simulink model "BPSK_Modulation"  (R2013a)
settings: Solver=ode3  StartTime=0.0  StopTime=0.06  FixedStep=1/(19200*2048)  RelTol=1e-3
libraries: simulink_extras x5, dsparch4 x2, simulink x1, commrandsrc2 x1
settings Model: Creator=Cedric  LastModifiedBy=Cedric
settings OptimizationCC: BooleanDataType=off

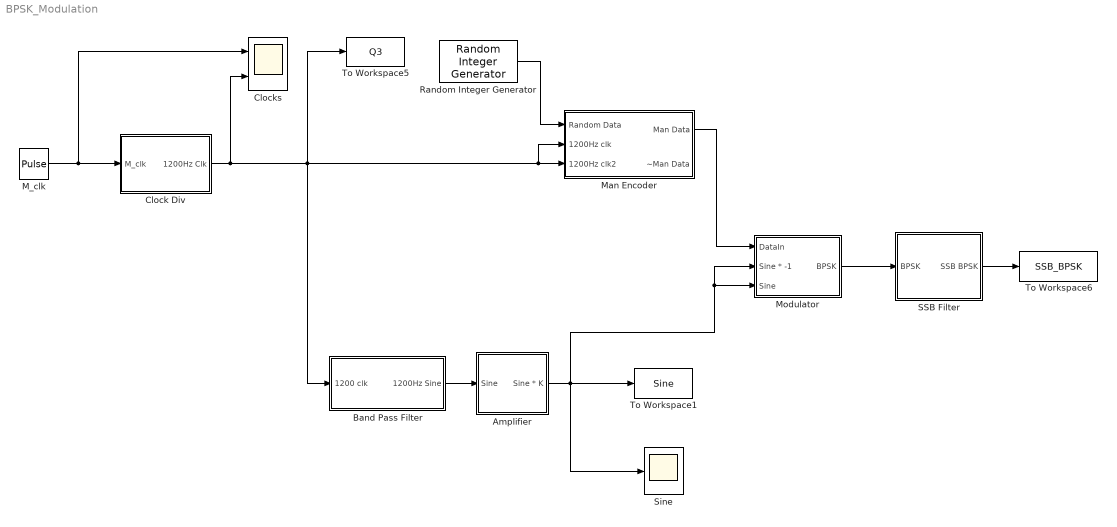
== system BPSK_Modulation ==
  Amplifier : Subsystem
  Band Pass Filter : Subsystem
  Clock Div : Subsystem
  Clocks : Scope  NumInputPorts=2
      settings: TimeRange=0.0003500000000000031  YMin=0~0  YMax=1~2
  M_clk : DiscretePulseGenerator  Period=4  PulseWidth=2  SampleTime=1/76800
  Man Encoder : Subsystem
  Modulator : Subsystem
  Random Integer Generator : commrandsrc2/Random Integer Generator  mul=2  seed=randseed  Ts=-1  frameBased=off  sampPerFrame=1  orient=on  outDataType=double
  SSB Filter : Subsystem
  Sine : Scope
  To Workspace1 : ToWorkspace  VariableName=Sine  SampleTime=-1  SaveFormat=Timeseries
  To Workspace5 : ToWorkspace  VariableName=Q3  SampleTime=-1  SaveFormat=Timeseries
  To Workspace6 : ToWorkspace  VariableName=SSB_BPSK  SampleTime=-1  SaveFormat=Timeseries
  wires:
  Amplifier/1(Sine * K) -> Sine/1, Modulator/2(Sine * -1), Modulator/3(Sine), To Workspace1/1
  Band Pass Filter/1(1200Hz Sine) -> Amplifier/1(Sine)
  Random Integer Generator/1 -> Man Encoder/1(Random Data)
  Man Encoder/1(Man Data) -> Modulator/1(DataIn)
  Modulator/1(BPSK) -> SSB Filter/1(BPSK)
  SSB Filter/1(SSB BPSK) -> To Workspace6/1
  Clock Div/1(1200Hz Clk) -> Clocks/2, Man Encoder/3("1200Hz clk2 "), Man Encoder/2(1200Hz clk), To Workspace5/1, Band Pass Filter/1(1200 clk)
  M_clk/1 -> Clocks/1, Clock Div/1(M_clk)

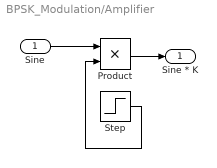
== system BPSK_Modulation/Amplifier ==
  Sine : Inport
  Product : Product
  Step : Step  Time=0
  Sine * K : Outport
  wires:
  Sine/1 -> Product/1
  Step/1 -> Product/2
  Product/1 -> Sine * K/1

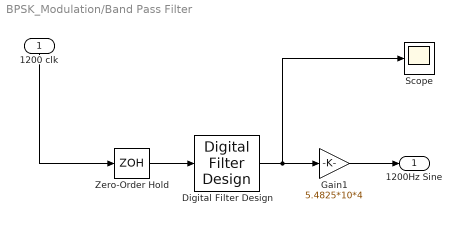
== system BPSK_Modulation/Band Pass Filter ==
  1200 clk : Inport
  Digital Filter Design : dsparch4/Digital Filter Design  mwdsp_browser_bugfix_var=off
  Gain1 : Gain  Gain=5.4825*10*4
  Scope : Scope
      settings: SaveName=ScopeData2
  Zero-Order Hold : ZeroOrderHold  SampleTime=-1
  1200Hz Sine : Outport
  wires:
  Zero-Order Hold/1 -> Digital Filter Design/1
  Digital Filter Design/1 -> Scope/1, Gain1/1
  1200 clk/1 -> Zero-Order Hold/1
  Gain1/1 -> 1200Hz Sine/1

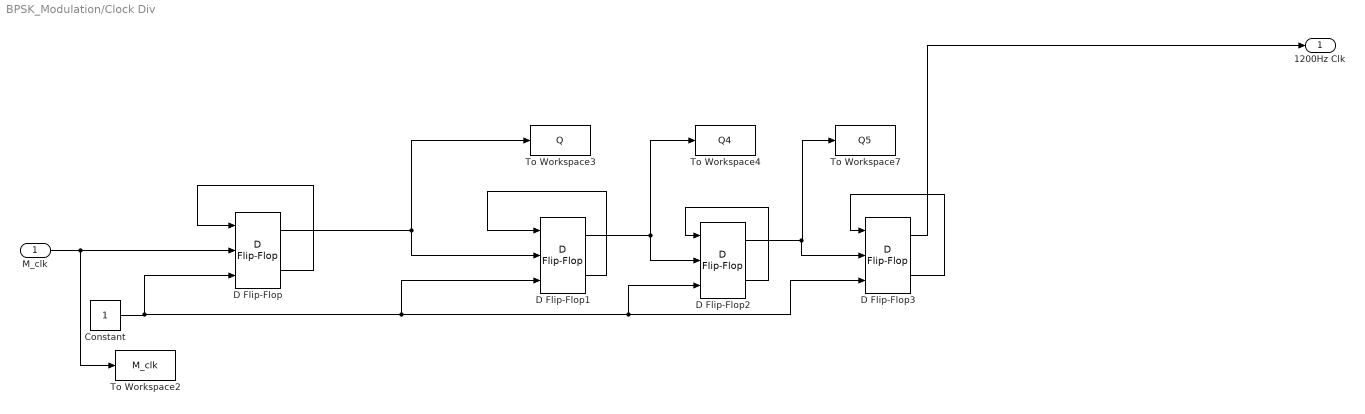
== system BPSK_Modulation/Clock Div ==
  M_clk : Inport
  Constant : Constant  SampleTime=-1
  D Flip-Flop{,1..3} (4 alike) : simulink_extras/Flip Flops/D Flip-Flop
  To Workspace2 : ToWorkspace  VariableName=M_clk  SampleTime=-1  SaveFormat=Timeseries
  To Workspace3 : ToWorkspace  VariableName=Q  SampleTime=-1  SaveFormat=Timeseries
  To Workspace4 : ToWorkspace  VariableName=Q4  SampleTime=-1  SaveFormat=Timeseries
  To Workspace7 : ToWorkspace  VariableName=Q5  SampleTime=-1  SaveFormat=Timeseries
  1200Hz Clk : Outport
  wires:
  D Flip-Flop3/1 -> 1200Hz Clk/1
  D Flip-Flop1/2 -> D Flip-Flop1/1
  D Flip-Flop/2 -> D Flip-Flop/1
  D Flip-Flop2/2 -> D Flip-Flop2/1
  Constant/1 -> D Flip-Flop3/3, D Flip-Flop2/3, D Flip-Flop1/3, D Flip-Flop/3
  D Flip-Flop3/2 -> D Flip-Flop3/1
  M_clk/1 -> To Workspace2/1, D Flip-Flop/2
  D Flip-Flop2/1 -> D Flip-Flop3/2, To Workspace7/1
  D Flip-Flop/1 -> To Workspace3/1, D Flip-Flop1/2
  D Flip-Flop1/1 -> To Workspace4/1, D Flip-Flop2/2

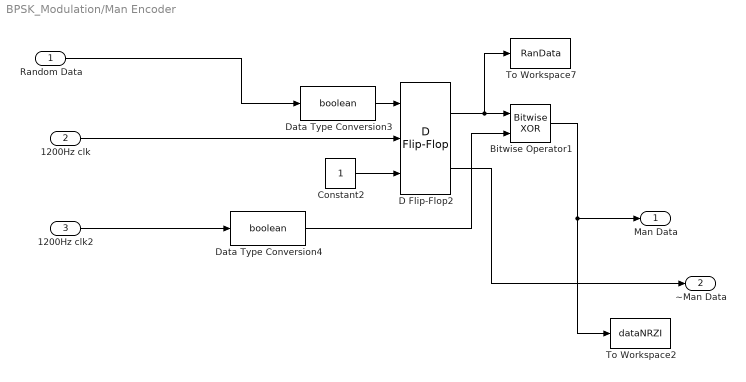
== system BPSK_Modulation/Man Encoder ==
  Random Data : Inport
  1200Hz clk : Inport  Port=2
  "1200Hz clk2 " : Inport  Port=3
  Bitwise Operator1 : simulink/Logic and Bit Operations/Bitwise Operator  logicop=XOR  UseBitMask=off  NumInputPorts=2  BitMask=bin2dec('11011001')  BitMaskRealWorld=Stored Integer
  Constant2 : Constant  SampleTime=-1
  D Flip-Flop2 : simulink_extras/Flip Flops/D Flip-Flop
  Data Type Conversion3 : DataTypeConversion  OutDataTypeStr=boolean
  Data Type Conversion4 : DataTypeConversion  OutDataTypeStr=boolean
  To Workspace2 : ToWorkspace  VariableName=dataNRZI  SampleTime=-1  SaveFormat=Timeseries
  To Workspace7 : ToWorkspace  VariableName=RanData  SampleTime=-1  SaveFormat=Timeseries
  Man Data : Outport
  ~Man Data : Outport  Port=2
  wires:
  D Flip-Flop2/1 -> To Workspace7/1, Bitwise Operator1/1
  Bitwise Operator1/1 -> Man Data/1, To Workspace2/1
  Data Type Conversion4/1 -> Bitwise Operator1/2
  D Flip-Flop2/2 -> ~Man Data/1
  "1200Hz clk2 "/1 -> Data Type Conversion4/1
  1200Hz clk/1 -> D Flip-Flop2/2
  Constant2/1 -> D Flip-Flop2/3
  Random Data/1 -> Data Type Conversion3/1
  Data Type Conversion3/1 -> D Flip-Flop2/1

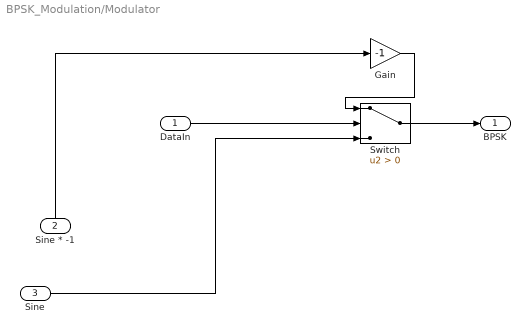
== system BPSK_Modulation/Modulator ==
  DataIn : Inport
  Sine * -1 : Inport  Port=2
  Sine : Inport  Port=3
  Gain : Gain  Gain=-1
  Switch : Switch  Criteria=u2 > Threshold
  BPSK : Outport
  wires:
  DataIn/1 -> Switch/2
  Sine/1 -> Switch/3
  Sine * -1/1 -> Gain/1
  Gain/1 -> Switch/1
  Switch/1 -> BPSK/1

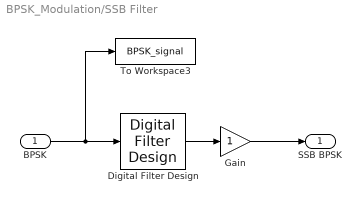
== system BPSK_Modulation/SSB Filter ==
  BPSK : Inport
  Digital Filter Design : dsparch4/Digital Filter Design  mwdsp_browser_bugfix_var=off
  Gain : Gain
  To Workspace3 : ToWorkspace  VariableName=BPSK_signal  SampleTime=-1  SaveFormat=Timeseries
  SSB BPSK : Outport
  wires:
  BPSK/1 -> Digital Filter Design/1, To Workspace3/1
  Digital Filter Design/1 -> Gain/1
  Gain/1 -> SSB BPSK/1
